simulink library "inp"  (R2021b)
settings: Solver=VariableStepAuto  StartTime=0.0  StopTime=10.0  RelTol=1e-3
undefined symbols (not defined in the file): C_TASK_5MS_S, FALSE, KINP_AcoreReadyToSlp_flg_ovrdflg, KINP_AcoreReadyToSlp_flg_ovrdval, KINP_AllowMovThd_OTA_enum_ovrdflg, KINP_AllowMovThd_OTA_enum_ovrdval, KINP_APSAngleTarget_Deg_ovrdflg, KINP_APSAngleTarget_Deg_ovrdval, KINP_APSDecReq_mps2_ovrdflg, KINP_APSDecReq_mps2_ovrdval, KINP_APSDecReqA_flg_ovrdflg, KINP_APSDecReqA_flg_ovrdval, KINP_APSDFLL_cm_ovrdflg, KINP_APSDFLL_cm_ovrdval, KINP_APSDFLR_cm_ovrdflg, KINP_APSDFLR_cm_ovrdval, KINP_APSDRLL_cm_ovrdflg, KINP_APSDRLL_cm_ovrdval, KINP_APSDRLR_cm_ovrdflg, KINP_APSDRLR_cm_ovrdval, KINP_APSExitCondition_enum_ovrdflg, KINP_APSExitCondition_enum_ovrdval, KINP_APSHWVer_enum_ovrdflg, KINP_APSHWVer_enum_ovrdval, KINP_APSProgressPCT_pct_ovrdflg, KINP_APSProgressPCT_pct_ovrdval, KINP_APSPwrReq_enum_ovrdflg, KINP_APSPwrReq_enum_ovrdval, KINP_APSReq_enum_ovrdflg, KINP_APSReq_enum_ovrdval, KINP_APSRQDisplay_enum_ovrdflg, KINP_APSRQDisplay_enum_ovrdval, KINP_APSRqEPASCtrl_flg_ovrdflg, KINP_APSRqEPASCtrl_flg_ovrdval, KINP_APSShiftPosnReq_enum_ovrdval, KINP_APSShiftPosnReq_enum_ovrflg, KINP_APSSpeedCMD_kph_ovrdval, KINP_APSSpeedCMD_kph_ovrflg, KINP_APSStaSystem_enum_ovrdflg, KINP_APSStaSystem_enum_ovrdval, KINP_APSSWVer_enum_ovrdflg, KINP_APSSWVer_enum_ovrdval, KINP_APSVMCReqA_flg_ovrdval, KINP_APSVMCReqA_flg_ovrflg, KINP_APSVRqEPASCtrl_flg_ovrdflg, KINP_APSVRqEPASCtrl_flg_ovrdval, KINP_AuxBattVolmV_mV_ovrdflg, KINP_AuxBattVolmV_mV_ovrdval, KINP_CAASSta_enum_ovrdflg, KINP_CAASSta_enum_ovrdval, KINP_CAASVMCReqA_flg_ovrdval, KINP_CAASVMCReqA_flg_ovrflg, KINP_CAN1BusOff_flg_ovrdflg, KINP_CAN1BusOff_flg_ovrdval, KINP_CAN2BusOff_flg_ovrdflg, KINP_CAN2BusOff_flg_ovrdval, KINP_CAN3BusOff_flg_ovrdflg, KINP_CAN3BusOff_flg_ovrdval, KINP_CAN4BusOff_flg_ovrdflg, KINP_CAN4BusOff_flg_ovrdval ... (+152)
libraries: FVT_lib x1035, hcu_lib x1
(part 23 of 33)

== system inp/INP/CAN3/SignalCheck/MCU_N_R1 ==
  BHAL_outputs : Inport
  inp_CanValid_bus : Inport  Port=2
  MCUNR1CSErr : FVT_lib/inp/can_signal_template  SystemSampleTime=-1  VariantActivationTime=update diagram  Latency=0  AutoFrameSizeCalculation=off
      link override defval: Value=KINP_MCUNR1CSErr_flg_defval
      link override ovrdflg: Value=KINP_MCUNR1CSErr_flg_ovrdflg
      link override ovrdval: Value=KINP_MCUNR1CSErr_flg_ovrdval
  MCUNR1RCErr : FVT_lib/inp/can_signal_template  SystemSampleTime=-1  VariantActivationTime=update diagram  Latency=0  AutoFrameSizeCalculation=off
      link override defval: Value=KINP_MCUNR1RCErr_flg_defval
      link override ovrdflg: Value=KINP_MCUNR1RCErr_flg_ovrdflg
      link override ovrdval: Value=KINP_MCUNR1RCErr_flg_ovrdval
  MCUWarnRNidec : FVT_lib/inp/can_signal_template  SystemSampleTime=-1  VariantActivationTime=update diagram  Latency=0  AutoFrameSizeCalculation=off
      link override defval: Value=KINP_MCUWarnRNidec_enum_defval
      link override ovrdflg: Value=KINP_MCUWarnRNidec_enum_ovrdflg
      link override ovrdval: Value=KINP_MCUWarnRNidec_enum_ovrdval
  RrActvDmpDisabStaNidec : FVT_lib/inp/can_signal_template  SystemSampleTime=-1  VariantActivationTime=update diagram  Latency=0  AutoFrameSizeCalculation=off
      link override defval: Value=KINP_RrActvDmpDisabStaNidec_flg_defval
      link override ovrdflg: Value=KINP_RrActvDmpDisabStaNidec_flg_ovrdflg
      link override ovrdval: Value=KINP_RrActvDmpDisabStaNidec_flg_ovrdval
  RrEDUDrtStaNidec : FVT_lib/inp/can_signal_template  SystemSampleTime=-1  VariantActivationTime=update diagram  Latency=0  AutoFrameSizeCalculation=off
      link override defval: Value=KINP_RrEDUDrtStaNidec_flg_defval
      link override ovrdflg: Value=KINP_RrEDUDrtStaNidec_flg_ovrdflg
      link override ovrdval: Value=KINP_RrEDUDrtStaNidec_flg_ovrdval
  RrEDUOpratingStaNidec : FVT_lib/inp/can_signal_template  SystemSampleTime=-1  VariantActivationTime=update diagram  Latency=0  AutoFrameSizeCalculation=off
      link override defval: Value=KINP_RrEDUOpratingStaNidec_flg_defval
      link override ovrdflg: Value=KINP_RrEDUOpratingStaNidec_flg_ovrdflg
      link override ovrdval: Value=KINP_RrEDUOpratingStaNidec_flg_ovrdval
  RrEDURealTMTqNidec : FVT_lib/inp/can_signal_template  SystemSampleTime=-1  VariantActivationTime=update diagram  Latency=0  AutoFrameSizeCalculation=off
      link override defval: Value=KINP_RrEDURealTMTqNidec_Nm_defval
      link override ovrdflg: Value=KINP_RrEDURealTMTqNidec_Nm_ovrdflg
      link override ovrdval: Value=KINP_RrEDURealTMTqNidec_Nm_ovrdval
  RrEDURotateDirctionNidec : FVT_lib/inp/can_signal_template  SystemSampleTime=-1  VariantActivationTime=update diagram  Latency=0  AutoFrameSizeCalculation=off
      link override defval: Value=KINP_RrEDURotateDirctionNidec_enum_defval
      link override ovrdflg: Value=KINP_RrEDURotateDirctionNidec_enum_ovrdflg
      link override ovrdval: Value=KINP_RrEDURotateDirctionNidec_enum_ovrdval
  RrEDUTqReqFbkNidec : FVT_lib/inp/can_signal_template  SystemSampleTime=-1  VariantActivationTime=update diagram  Latency=0  AutoFrameSizeCalculation=off
      link override defval: Value=KINP_RrEDUTqReqFbkNidec_Nm_defval
      link override ovrdflg: Value=KINP_RrEDUTqReqFbkNidec_Nm_ovrdflg
      link override ovrdval: Value=KINP_RrEDUTqReqFbkNidec_Nm_ovrdval
  RrMCU1ChksumNidec : FVT_lib/inp/can_signal_template  SystemSampleTime=-1  VariantActivationTime=update diagram  Latency=0  AutoFrameSizeCalculation=off
      link override defval: Value=KINP_RrMCU1ChksumNidec_enum_defval
      link override ovrdflg: Value=KINP_RrMCU1ChksumNidec_enum_ovrdflg
      link override ovrdval: Value=KINP_RrMCU1ChksumNidec_enum_ovrdval
  RrMCU1RolCntNidec : FVT_lib/inp/can_signal_template  SystemSampleTime=-1  VariantActivationTime=update diagram  Latency=0  AutoFrameSizeCalculation=off
      link override defval: Value=KINP_RrMCU1RolCntNidec_enum_defval
      link override ovrdflg: Value=KINP_RrMCU1RolCntNidec_enum_ovrdflg
      link override ovrdval: Value=KINP_RrMCU1RolCntNidec_enum_ovrdval
  RrMCUBATNidec : FVT_lib/inp/can_signal_template  SystemSampleTime=-1  VariantActivationTime=update diagram  Latency=0  AutoFrameSizeCalculation=off
      link override defval: Value=KINP_RrMCUBATNidec_V_defval
      link override ovrdflg: Value=KINP_RrMCUBATNidec_V_ovrdflg
      link override ovrdval: Value=KINP_RrMCUBATNidec_V_ovrdval
  RrMCUDCBusCurrNidec : FVT_lib/inp/can_signal_template  SystemSampleTime=-1  VariantActivationTime=update diagram  Latency=0  AutoFrameSizeCalculation=off
      link override defval: Value=KINP_RrMCUDCBusCurrNidec_A_defval
      link override ovrdflg: Value=KINP_RrMCUDCBusCurrNidec_A_ovrdflg
      link override ovrdval: Value=KINP_RrMCUDCBusCurrNidec_A_ovrdval
  RrMCUDCBusVoltNidec : FVT_lib/inp/can_signal_template  SystemSampleTime=-1  VariantActivationTime=update diagram  Latency=0  AutoFrameSizeCalculation=off
      link override defval: Value=KINP_RrMCUDCBusVoltNidec_V_defval
      link override ovrdflg: Value=KINP_RrMCUDCBusVoltNidec_V_ovrdflg
      link override ovrdval: Value=KINP_RrMCUDCBusVoltNidec_V_ovrdval
  RrMCUDischrgStaNidec : FVT_lib/inp/can_signal_template  SystemSampleTime=-1  VariantActivationTime=update diagram  Latency=0  AutoFrameSizeCalculation=off
      link override defval: Value=KINP_RrMCUDischrgStaNidec_flg_defval
      link override ovrdflg: Value=KINP_RrMCUDischrgStaNidec_flg_ovrdflg
      link override ovrdval: Value=KINP_RrMCUDischrgStaNidec_flg_ovrdval
  RrMCUEnaStaNidec : FVT_lib/inp/can_signal_template  SystemSampleTime=-1  VariantActivationTime=update diagram  Latency=0  AutoFrameSizeCalculation=off
      link override defval: Value=KINP_RrMCUEnaStaNidec_flg_defval
      link override ovrdflg: Value=KINP_RrMCUEnaStaNidec_flg_ovrdflg
      link override ovrdval: Value=KINP_RrMCUEnaStaNidec_flg_ovrdval
  RrMCUErrNidec : FVT_lib/inp/can_signal_template  SystemSampleTime=-1  VariantActivationTime=update diagram  Latency=0  AutoFrameSizeCalculation=off
      link override defval: Value=KINP_RrMCUErrNidec_enum_defval
      link override ovrdflg: Value=KINP_RrMCUErrNidec_enum_ovrdflg
      link override ovrdval: Value=KINP_RrMCUErrNidec_enum_ovrdval
  RrMCUIGNstaNidec : FVT_lib/inp/can_signal_template  SystemSampleTime=-1  VariantActivationTime=update diagram  Latency=0  AutoFrameSizeCalculation=off
      link override defval: Value=KINP_RrMCUIGNstaNidec_flg_defval
      link override ovrdflg: Value=KINP_RrMCUIGNstaNidec_flg_ovrdflg
      link override ovrdval: Value=KINP_RrMCUIGNstaNidec_flg_ovrdval
  RrMCUReady4PreNidec : FVT_lib/inp/can_signal_template  SystemSampleTime=-1  VariantActivationTime=update diagram  Latency=0  AutoFrameSizeCalculation=off
      link override defval: Value=KINP_RrMCUReady4PreNidec_flg_defval
      link override ovrdflg: Value=KINP_RrMCUReady4PreNidec_flg_ovrdflg
      link override ovrdval: Value=KINP_RrMCUReady4PreNidec_flg_ovrdval
  RrMCUReadyNidec : FVT_lib/inp/can_signal_template  SystemSampleTime=-1  VariantActivationTime=update diagram  Latency=0  AutoFrameSizeCalculation=off
      link override defval: Value=KINP_RrMCUReadyNidec_flg_defval
      link override ovrdflg: Value=KINP_RrMCUReadyNidec_flg_ovrdflg
      link override ovrdval: Value=KINP_RrMCUReadyNidec_flg_ovrdval
  RrMCUSysStaNidec : FVT_lib/inp/can_signal_template  SystemSampleTime=-1  VariantActivationTime=update diagram  Latency=0  AutoFrameSizeCalculation=off
      link override defval: Value=KINP_RrMCUSysStaNidec_enum_defval
      link override ovrdflg: Value=KINP_RrMCUSysStaNidec_enum_ovrdflg
      link override ovrdval: Value=KINP_RrMCUSysStaNidec_enum_ovrdval
  RrMCUTempNidec : FVT_lib/inp/can_signal_template  SystemSampleTime=-1  VariantActivationTime=update diagram  Latency=0  AutoFrameSizeCalculation=off
      link override defval: Value=KINP_RrMCUTempNidec_C_defval
      link override ovrdflg: Value=KINP_RrMCUTempNidec_C_ovrdflg
      link override ovrdval: Value=KINP_RrMCUTempNidec_C_ovrdval
  RrMotorAvailTqNidec : FVT_lib/inp/can_signal_template  SystemSampleTime=-1  VariantActivationTime=update diagram  Latency=0  AutoFrameSizeCalculation=off
      link override defval: Value=KINP_RrMotorAvailTqNidec_Nm_defval
      link override ovrdflg: Value=KINP_RrMotorAvailTqNidec_Nm_ovrdflg
      link override ovrdval: Value=KINP_RrMotorAvailTqNidec_Nm_ovrdval
  RrRegenAvailTqNidec : FVT_lib/inp/can_signal_template  SystemSampleTime=-1  VariantActivationTime=update diagram  Latency=0  AutoFrameSizeCalculation=off
      link override defval: Value=KINP_RrRegenAvailTqNidec_Nm_defval
      link override ovrdflg: Value=KINP_RrRegenAvailTqNidec_Nm_ovrdflg
      link override ovrdval: Value=KINP_RrRegenAvailTqNidec_Nm_ovrdval
  RrTMSpdNidec : FVT_lib/inp/can_signal_template  SystemSampleTime=-1  VariantActivationTime=update diagram  Latency=0  AutoFrameSizeCalculation=off
      link override defval: Value=KINP_RrTMSpdNidec_rpm_defval
      link override ovrdflg: Value=KINP_RrTMSpdNidec_rpm_ovrdflg
      link override ovrdval: Value=KINP_RrTMSpdNidec_rpm_ovrdval
  RrTMTempNidec : FVT_lib/inp/can_signal_template  SystemSampleTime=-1  VariantActivationTime=update diagram  Latency=0  AutoFrameSizeCalculation=off
      link override defval: Value=KINP_RrTMTempNidec_C_defval
      link override ovrdflg: Value=KINP_RrTMTempNidec_C_ovrdflg
      link override ovrdval: Value=KINP_RrTMTempNidec_C_ovrdval
  RrTMidNidec : FVT_lib/inp/can_signal_template  SystemSampleTime=-1  VariantActivationTime=update diagram  Latency=0  AutoFrameSizeCalculation=off
      link override defval: Value=KINP_RrTMidNidec_A_defval
      link override ovrdflg: Value=KINP_RrTMidNidec_A_ovrdflg
      link override ovrdval: Value=KINP_RrTMidNidec_A_ovrdval
  RrTMiqNidec : FVT_lib/inp/can_signal_template  SystemSampleTime=-1  VariantActivationTime=update diagram  Latency=0  AutoFrameSizeCalculation=off
      link override defval: Value=KINP_RrTMiqNidec_A_defval
      link override ovrdflg: Value=KINP_RrTMiqNidec_A_ovrdflg
      link override ovrdval: Value=KINP_RrTMiqNidec_A_ovrdval
  Terminator_{1..28} (28 alike) : Terminator
  True_VHAL_MCUNR1CSErr_flg : Constant  Value=TRUE  OutDataTypeStr=boolean
  True_VHAL_MCUNR1RCErr_flg : Constant  Value=TRUE  OutDataTypeStr=boolean
  True_VHAL_MCUWarnRNidec_enum : Constant  Value=TRUE  OutDataTypeStr=boolean
  True_VHAL_RrActvDmpDisabStaNidec_flg : Constant  Value=TRUE  OutDataTypeStr=boolean
  True_VHAL_RrEDUDrtStaNidec_flg : Constant  Value=TRUE  OutDataTypeStr=boolean
  True_VHAL_RrEDUOpratingStaNidec_flg : Constant  Value=TRUE  OutDataTypeStr=boolean
  True_VHAL_RrEDURealTMTqNidec_Nm : Constant  Value=TRUE  OutDataTypeStr=boolean
  True_VHAL_RrEDURotateDirctionNidec_enum : Constant  Value=TRUE  OutDataTypeStr=boolean
  True_VHAL_RrEDUTqReqFbkNidec_Nm : Constant  Value=TRUE  OutDataTypeStr=boolean
  True_VHAL_RrMCU1ChksumNidec_enum : Constant  Value=TRUE  OutDataTypeStr=boolean
  True_VHAL_RrMCU1RolCntNidec_enum : Constant  Value=TRUE  OutDataTypeStr=boolean
  True_VHAL_RrMCUBATNidec_V : Constant  Value=TRUE  OutDataTypeStr=boolean
  True_VHAL_RrMCUDCBusCurrNidec_A : Constant  Value=TRUE  OutDataTypeStr=boolean
  True_VHAL_RrMCUDCBusVoltNidec_V : Constant  Value=TRUE  OutDataTypeStr=boolean
  True_VHAL_RrMCUDischrgStaNidec_flg : Constant  Value=TRUE  OutDataTypeStr=boolean
  True_VHAL_RrMCUEnaStaNidec_flg : Constant  Value=TRUE  OutDataTypeStr=boolean
  True_VHAL_RrMCUErrNidec_enum : Constant  Value=TRUE  OutDataTypeStr=boolean
  True_VHAL_RrMCUIGNstaNidec_flg : Constant  Value=TRUE  OutDataTypeStr=boolean
  True_VHAL_RrMCUReady4PreNidec_flg : Constant  Value=TRUE  OutDataTypeStr=boolean
  True_VHAL_RrMCUReadyNidec_flg : Constant  Value=TRUE  OutDataTypeStr=boolean
  True_VHAL_RrMCUSysStaNidec_enum : Constant  Value=TRUE  OutDataTypeStr=boolean
  True_VHAL_RrMCUTempNidec_C : Constant  Value=TRUE  OutDataTypeStr=boolean
  True_VHAL_RrMotorAvailTqNidec_Nm : Constant  Value=TRUE  OutDataTypeStr=boolean
  True_VHAL_RrRegenAvailTqNidec_Nm : Constant  Value=TRUE  OutDataTypeStr=boolean
  True_VHAL_RrTMSpdNidec_rpm : Constant  Value=TRUE  OutDataTypeStr=boolean
  True_VHAL_RrTMTempNidec_C : Constant  Value=TRUE  OutDataTypeStr=boolean
  True_VHAL_RrTMidNidec_A : Constant  Value=TRUE  OutDataTypeStr=boolean
  True_VHAL_RrTMiqNidec_A : Constant  Value=TRUE  OutDataTypeStr=boolean
  slr1_{1..28} (28 alike) : BusSelector  OutputSignals=VINP_CANMsgValidMCUNR1_flg
  slr_VHAL_MCUNR1CSErr_flg : BusSelector  OutputSignals=VHAL_MCUNR1CSErr_flg
  slr_VHAL_MCUNR1RCErr_flg : BusSelector  OutputSignals=VHAL_MCUNR1RCErr_flg
  slr_VHAL_MCUWarnRNidec_enum : BusSelector  OutputSignals=VHAL_MCUWarnRNidec_enum
  slr_VHAL_RrActvDmpDisabStaNidec_flg : BusSelector  OutputSignals=VHAL_RrActvDmpDisabStaNidec_flg
  slr_VHAL_RrEDUDrtStaNidec_flg : BusSelector  OutputSignals=VHAL_RrEDUDrtStaNidec_flg
  slr_VHAL_RrEDUOpratingStaNidec_flg : BusSelector  OutputSignals=VHAL_RrEDUOpratingStaNidec_flg
  slr_VHAL_RrEDURealTMTqNidec_Nm : BusSelector  OutputSignals=VHAL_RrEDURealTMTqNidec_Nm
  slr_VHAL_RrEDURotateDirctionNidec_enum : BusSelector  OutputSignals=VHAL_RrEDURotateDirctionNidec_enum
  slr_VHAL_RrEDUTqReqFbkNidec_Nm : BusSelector  OutputSignals=VHAL_RrEDUTqReqFbkNidec_Nm
  slr_VHAL_RrMCU1ChksumNidec_enum : BusSelector  OutputSignals=VHAL_RrMCU1ChksumNidec_enum
  slr_VHAL_RrMCU1RolCntNidec_enum : BusSelector  OutputSignals=VHAL_RrMCU1RolCntNidec_enum
  slr_VHAL_RrMCUBATNidec_V : BusSelector  OutputSignals=VHAL_RrMCUBATNidec_V
  slr_VHAL_RrMCUDCBusCurrNidec_A : BusSelector  OutputSignals=VHAL_RrMCUDCBusCurrNidec_A
  slr_VHAL_RrMCUDCBusVoltNidec_V : BusSelector  OutputSignals=VHAL_RrMCUDCBusVoltNidec_V
  slr_VHAL_RrMCUDischrgStaNidec_flg : BusSelector  OutputSignals=VHAL_RrMCUDischrgStaNidec_flg
  slr_VHAL_RrMCUEnaStaNidec_flg : BusSelector  OutputSignals=VHAL_RrMCUEnaStaNidec_flg
  slr_VHAL_RrMCUErrNidec_enum : BusSelector  OutputSignals=VHAL_RrMCUErrNidec_enum
  slr_VHAL_RrMCUIGNstaNidec_flg : BusSelector  OutputSignals=VHAL_RrMCUIGNstaNidec_flg
  slr_VHAL_RrMCUReady4PreNidec_flg : BusSelector  OutputSignals=VHAL_RrMCUReady4PreNidec_flg
  slr_VHAL_RrMCUReadyNidec_flg : BusSelector  OutputSignals=VHAL_RrMCUReadyNidec_flg
  slr_VHAL_RrMCUSysStaNidec_enum : BusSelector  OutputSignals=VHAL_RrMCUSysStaNidec_enum
  slr_VHAL_RrMCUTempNidec_C : BusSelector  OutputSignals=VHAL_RrMCUTempNidec_C
  slr_VHAL_RrMotorAvailTqNidec_Nm : BusSelector  OutputSignals=VHAL_RrMotorAvailTqNidec_Nm
  slr_VHAL_RrRegenAvailTqNidec_Nm : BusSelector  OutputSignals=VHAL_RrRegenAvailTqNidec_Nm
  slr_VHAL_RrTMSpdNidec_rpm : BusSelector  OutputSignals=VHAL_RrTMSpdNidec_rpm
  slr_VHAL_RrTMTempNidec_C : BusSelector  OutputSignals=VHAL_RrTMTempNidec_C
  slr_VHAL_RrTMidNidec_A : BusSelector  OutputSignals=VHAL_RrTMidNidec_A
  slr_VHAL_RrTMiqNidec_A : BusSelector  OutputSignals=VHAL_RrTMiqNidec_A
  VINP_MCUNR1CSErr_flg : Outport
  VINP_MCUNR1RCErr_flg : Outport  Port=2
  VINP_MCUWarnRNidec_enum : Outport  Port=3
  VINP_RrActvDmpDisabStaNidec_flg : Outport  Port=4
  VINP_RrEDUDrtStaNidec_flg : Outport  Port=5
  VINP_RrEDUOpratingStaNidec_flg : Outport  Port=6
  VINP_RrEDURealTMTqNidec_Nm : Outport  Port=7
  VINP_RrEDURotateDirctionNidec_enum : Outport  Port=8
  VINP_RrEDUTqReqFbkNidec_Nm : Outport  Port=9
  VINP_RrMCU1ChksumNidec_enum : Outport  Port=10
  VINP_RrMCU1RolCntNidec_enum : Outport  Port=11
  VINP_RrMCUBATNidec_V : Outport  Port=12
  VINP_RrMCUDCBusCurrNidec_A : Outport  Port=13
  VINP_RrMCUDCBusVoltNidec_V : Outport  Port=14
  VINP_RrMCUDischrgStaNidec_flg : Outport  Port=15
  VINP_RrMCUEnaStaNidec_flg : Outport  Port=16
  VINP_RrMCUErrNidec_enum : Outport  Port=17
  VINP_RrMCUIGNstaNidec_flg : Outport  Port=18
  VINP_RrMCUReady4PreNidec_flg : Outport  Port=19
  VINP_RrMCUReadyNidec_flg : Outport  Port=20
  VINP_RrMCUSysStaNidec_enum : Outport  Port=21
  VINP_RrMCUTempNidec_C : Outport  Port=22
  VINP_RrMotorAvailTqNidec_Nm : Outport  Port=23
  VINP_RrRegenAvailTqNidec_Nm : Outport  Port=24
  VINP_RrTMSpdNidec_rpm : Outport  Port=25
  VINP_RrTMTempNidec_C : Outport  Port=26
  VINP_RrTMidNidec_A : Outport  Port=27
  VINP_RrTMiqNidec_A : Outport  Port=28
  wires:
  BHAL_outputs/1 -> [BHAL_outputs]
  inp_CanValid_bus/1 -> [inp_CanValid_bus]
  [BHAL_outputs] -> slr_VHAL_MCUNR1CSErr_flg/1
  slr_VHAL_MCUNR1CSErr_flg/1 -> MCUNR1CSErr/1  "<VHAL_MCUNR1CSErr_flg>"
  True_VHAL_MCUNR1CSErr_flg/1 -> MCUNR1CSErr/2
  [inp_CanValid_bus] -> slr1_1/1
  slr1_1/1 -> MCUNR1CSErr/3  "<VINP_CANMsgValidMCUNR1_flg>"
  MCUNR1CSErr/1 -> VINP_MCUNR1CSErr_flg/1  "VINP_MCUNR1CSErr_flg"
  MCUNR1CSErr/2 -> Terminator_1/1
  [BHAL_outputs] -> slr_VHAL_MCUNR1RCErr_flg/1
  slr_VHAL_MCUNR1RCErr_flg/1 -> MCUNR1RCErr/1  "<VHAL_MCUNR1RCErr_flg>"
  True_VHAL_MCUNR1RCErr_flg/1 -> MCUNR1RCErr/2
  [inp_CanValid_bus] -> slr1_2/1
  slr1_2/1 -> MCUNR1RCErr/3  "<VINP_CANMsgValidMCUNR1_flg>"
  MCUNR1RCErr/1 -> VINP_MCUNR1RCErr_flg/1  "VINP_MCUNR1RCErr_flg"
  MCUNR1RCErr/2 -> Terminator_2/1
  [BHAL_outputs] -> slr_VHAL_MCUWarnRNidec_enum/1
  slr_VHAL_MCUWarnRNidec_enum/1 -> MCUWarnRNidec/1  "<VHAL_MCUWarnRNidec_enum>"
  True_VHAL_MCUWarnRNidec_enum/1 -> MCUWarnRNidec/2
  [inp_CanValid_bus] -> slr1_3/1
  slr1_3/1 -> MCUWarnRNidec/3  "<VINP_CANMsgValidMCUNR1_flg>"
  MCUWarnRNidec/1 -> VINP_MCUWarnRNidec_enum/1  "VINP_MCUWarnRNidec_enum"
  MCUWarnRNidec/2 -> Terminator_3/1
  [BHAL_outputs] -> slr_VHAL_RrActvDmpDisabStaNidec_flg/1
  slr_VHAL_RrActvDmpDisabStaNidec_flg/1 -> RrActvDmpDisabStaNidec/1  "<VHAL_RrActvDmpDisabStaNidec_flg>"
  True_VHAL_RrActvDmpDisabStaNidec_flg/1 -> RrActvDmpDisabStaNidec/2
  [inp_CanValid_bus] -> slr1_4/1
  slr1_4/1 -> RrActvDmpDisabStaNidec/3  "<VINP_CANMsgValidMCUNR1_flg>"
  RrActvDmpDisabStaNidec/1 -> VINP_RrActvDmpDisabStaNidec_flg/1  "VINP_RrActvDmpDisabStaNidec_flg"
  RrActvDmpDisabStaNidec/2 -> Terminator_4/1
  [BHAL_outputs] -> slr_VHAL_RrEDUDrtStaNidec_flg/1
  slr_VHAL_RrEDUDrtStaNidec_flg/1 -> RrEDUDrtStaNidec/1  "<VHAL_RrEDUDrtStaNidec_flg>"
  True_VHAL_RrEDUDrtStaNidec_flg/1 -> RrEDUDrtStaNidec/2
  [inp_CanValid_bus] -> slr1_5/1
  slr1_5/1 -> RrEDUDrtStaNidec/3  "<VINP_CANMsgValidMCUNR1_flg>"
  RrEDUDrtStaNidec/1 -> VINP_RrEDUDrtStaNidec_flg/1  "VINP_RrEDUDrtStaNidec_flg"
  RrEDUDrtStaNidec/2 -> Terminator_5/1
  [BHAL_outputs] -> slr_VHAL_RrEDUOpratingStaNidec_flg/1
  slr_VHAL_RrEDUOpratingStaNidec_flg/1 -> RrEDUOpratingStaNidec/1  "<VHAL_RrEDUOpratingStaNidec_flg>"
  True_VHAL_RrEDUOpratingStaNidec_flg/1 -> RrEDUOpratingStaNidec/2
  [inp_CanValid_bus] -> slr1_6/1
  slr1_6/1 -> RrEDUOpratingStaNidec/3  "<VINP_CANMsgValidMCUNR1_flg>"
  RrEDUOpratingStaNidec/1 -> VINP_RrEDUOpratingStaNidec_flg/1  "VINP_RrEDUOpratingStaNidec_flg"
  RrEDUOpratingStaNidec/2 -> Terminator_6/1
  [BHAL_outputs] -> slr_VHAL_RrEDURealTMTqNidec_Nm/1
  slr_VHAL_RrEDURealTMTqNidec_Nm/1 -> RrEDURealTMTqNidec/1  "<VHAL_RrEDURealTMTqNidec_Nm>"
  True_VHAL_RrEDURealTMTqNidec_Nm/1 -> RrEDURealTMTqNidec/2
  [inp_CanValid_bus] -> slr1_7/1
  slr1_7/1 -> RrEDURealTMTqNidec/3  "<VINP_CANMsgValidMCUNR1_flg>"
  RrEDURealTMTqNidec/1 -> VINP_RrEDURealTMTqNidec_Nm/1  "VINP_RrEDURealTMTqNidec_Nm"
  RrEDURealTMTqNidec/2 -> Terminator_7/1
  [BHAL_outputs] -> slr_VHAL_RrEDURotateDirctionNidec_enum/1
  slr_VHAL_RrEDURotateDirctionNidec_enum/1 -> RrEDURotateDirctionNidec/1  "<VHAL_RrEDURotateDirctionNidec_enum>"
  True_VHAL_RrEDURotateDirctionNidec_enum/1 -> RrEDURotateDirctionNidec/2
  [inp_CanValid_bus] -> slr1_8/1
  slr1_8/1 -> RrEDURotateDirctionNidec/3  "<VINP_CANMsgValidMCUNR1_flg>"
  RrEDURotateDirctionNidec/1 -> VINP_RrEDURotateDirctionNidec_enum/1  "VINP_RrEDURotateDirctionNidec_enum"
  RrEDURotateDirctionNidec/2 -> Terminator_8/1
  [BHAL_outputs] -> slr_VHAL_RrEDUTqReqFbkNidec_Nm/1
  slr_VHAL_RrEDUTqReqFbkNidec_Nm/1 -> RrEDUTqReqFbkNidec/1  "<VHAL_RrEDUTqReqFbkNidec_Nm>"
  True_VHAL_RrEDUTqReqFbkNidec_Nm/1 -> RrEDUTqReqFbkNidec/2
  [inp_CanValid_bus] -> slr1_9/1
  slr1_9/1 -> RrEDUTqReqFbkNidec/3  "<VINP_CANMsgValidMCUNR1_flg>"
  RrEDUTqReqFbkNidec/1 -> VINP_RrEDUTqReqFbkNidec_Nm/1  "VINP_RrEDUTqReqFbkNidec_Nm"
  RrEDUTqReqFbkNidec/2 -> Terminator_9/1
  [BHAL_outputs] -> slr_VHAL_RrMCU1ChksumNidec_enum/1
  slr_VHAL_RrMCU1ChksumNidec_enum/1 -> RrMCU1ChksumNidec/1  "<VHAL_RrMCU1ChksumNidec_enum>"
  True_VHAL_RrMCU1ChksumNidec_enum/1 -> RrMCU1ChksumNidec/2
  [inp_CanValid_bus] -> slr1_10/1
  slr1_10/1 -> RrMCU1ChksumNidec/3  "<VINP_CANMsgValidMCUNR1_flg>"
  RrMCU1ChksumNidec/1 -> VINP_RrMCU1ChksumNidec_enum/1  "VINP_RrMCU1ChksumNidec_enum"
  RrMCU1ChksumNidec/2 -> Terminator_10/1
  [BHAL_outputs] -> slr_VHAL_RrMCU1RolCntNidec_enum/1
  slr_VHAL_RrMCU1RolCntNidec_enum/1 -> RrMCU1RolCntNidec/1  "<VHAL_RrMCU1RolCntNidec_enum>"
  True_VHAL_RrMCU1RolCntNidec_enum/1 -> RrMCU1RolCntNidec/2
  [inp_CanValid_bus] -> slr1_11/1
  slr1_11/1 -> RrMCU1RolCntNidec/3  "<VINP_CANMsgValidMCUNR1_flg>"
  RrMCU1RolCntNidec/1 -> VINP_RrMCU1RolCntNidec_enum/1  "VINP_RrMCU1RolCntNidec_enum"
  RrMCU1RolCntNidec/2 -> Terminator_11/1
  [BHAL_outputs] -> slr_VHAL_RrMCUBATNidec_V/1
  slr_VHAL_RrMCUBATNidec_V/1 -> RrMCUBATNidec/1  "<VHAL_RrMCUBATNidec_V>"
  True_VHAL_RrMCUBATNidec_V/1 -> RrMCUBATNidec/2
  [inp_CanValid_bus] -> slr1_12/1
  slr1_12/1 -> RrMCUBATNidec/3  "<VINP_CANMsgValidMCUNR1_flg>"
  RrMCUBATNidec/1 -> VINP_RrMCUBATNidec_V/1  "VINP_RrMCUBATNidec_V"
  RrMCUBATNidec/2 -> Terminator_12/1
  [BHAL_outputs] -> slr_VHAL_RrMCUDCBusCurrNidec_A/1
  slr_VHAL_RrMCUDCBusCurrNidec_A/1 -> RrMCUDCBusCurrNidec/1  "<VHAL_RrMCUDCBusCurrNidec_A>"
  True_VHAL_RrMCUDCBusCurrNidec_A/1 -> RrMCUDCBusCurrNidec/2
  [inp_CanValid_bus] -> slr1_13/1
  slr1_13/1 -> RrMCUDCBusCurrNidec/3  "<VINP_CANMsgValidMCUNR1_flg>"
  RrMCUDCBusCurrNidec/1 -> VINP_RrMCUDCBusCurrNidec_A/1  "VINP_RrMCUDCBusCurrNidec_A"
  RrMCUDCBusCurrNidec/2 -> Terminator_13/1
  [BHAL_outputs] -> slr_VHAL_RrMCUDCBusVoltNidec_V/1
  slr_VHAL_RrMCUDCBusVoltNidec_V/1 -> RrMCUDCBusVoltNidec/1  "<VHAL_RrMCUDCBusVoltNidec_V>"
  True_VHAL_RrMCUDCBusVoltNidec_V/1 -> RrMCUDCBusVoltNidec/2
  [inp_CanValid_bus] -> slr1_14/1
  slr1_14/1 -> RrMCUDCBusVoltNidec/3  "<VINP_CANMsgValidMCUNR1_flg>"
  RrMCUDCBusVoltNidec/1 -> VINP_RrMCUDCBusVoltNidec_V/1  "VINP_RrMCUDCBusVoltNidec_V"
  RrMCUDCBusVoltNidec/2 -> Terminator_14/1
  [BHAL_outputs] -> slr_VHAL_RrMCUDischrgStaNidec_flg/1
  slr_VHAL_RrMCUDischrgStaNidec_flg/1 -> RrMCUDischrgStaNidec/1  "<VHAL_RrMCUDischrgStaNidec_flg>"
  True_VHAL_RrMCUDischrgStaNidec_flg/1 -> RrMCUDischrgStaNidec/2
  [inp_CanValid_bus] -> slr1_15/1
  slr1_15/1 -> RrMCUDischrgStaNidec/3  "<VINP_CANMsgValidMCUNR1_flg>"
  RrMCUDischrgStaNidec/1 -> VINP_RrMCUDischrgStaNidec_flg/1  "VINP_RrMCUDischrgStaNidec_flg"
  RrMCUDischrgStaNidec/2 -> Terminator_15/1
  [BHAL_outputs] -> slr_VHAL_RrMCUEnaStaNidec_flg/1
  slr_VHAL_RrMCUEnaStaNidec_flg/1 -> RrMCUEnaStaNidec/1  "<VHAL_RrMCUEnaStaNidec_flg>"
  True_VHAL_RrMCUEnaStaNidec_flg/1 -> RrMCUEnaStaNidec/2
  [inp_CanValid_bus] -> slr1_16/1
  slr1_16/1 -> RrMCUEnaStaNidec/3  "<VINP_CANMsgValidMCUNR1_flg>"
  RrMCUEnaStaNidec/1 -> VINP_RrMCUEnaStaNidec_flg/1  "VINP_RrMCUEnaStaNidec_flg"
  RrMCUEnaStaNidec/2 -> Terminator_16/1
  [BHAL_outputs] -> slr_VHAL_RrMCUErrNidec_enum/1
  slr_VHAL_RrMCUErrNidec_enum/1 -> RrMCUErrNidec/1  "<VHAL_RrMCUErrNidec_enum>"
  True_VHAL_RrMCUErrNidec_enum/1 -> RrMCUErrNidec/2
  [inp_CanValid_bus] -> slr1_17/1
  slr1_17/1 -> RrMCUErrNidec/3  "<VINP_CANMsgValidMCUNR1_flg>"
  RrMCUErrNidec/1 -> VINP_RrMCUErrNidec_enum/1  "VINP_RrMCUErrNidec_enum"
  RrMCUErrNidec/2 -> Terminator_17/1
  [BHAL_outputs] -> slr_VHAL_RrMCUIGNstaNidec_flg/1
  slr_VHAL_RrMCUIGNstaNidec_flg/1 -> RrMCUIGNstaNidec/1  "<VHAL_RrMCUIGNstaNidec_flg>"
  True_VHAL_RrMCUIGNstaNidec_flg/1 -> RrMCUIGNstaNidec/2
  [inp_CanValid_bus] -> slr1_18/1
  slr1_18/1 -> RrMCUIGNstaNidec/3  "<VINP_CANMsgValidMCUNR1_flg>"
  RrMCUIGNstaNidec/1 -> VINP_RrMCUIGNstaNidec_flg/1  "VINP_RrMCUIGNstaNidec_flg"
  RrMCUIGNstaNidec/2 -> Terminator_18/1
  [BHAL_outputs] -> slr_VHAL_RrMCUReady4PreNidec_flg/1
  slr_VHAL_RrMCUReady4PreNidec_flg/1 -> RrMCUReady4PreNidec/1  "<VHAL_RrMCUReady4PreNidec_flg>"
  True_VHAL_RrMCUReady4PreNidec_flg/1 -> RrMCUReady4PreNidec/2
  [inp_CanValid_bus] -> slr1_19/1
  slr1_19/1 -> RrMCUReady4PreNidec/3  "<VINP_CANMsgValidMCUNR1_flg>"
  RrMCUReady4PreNidec/1 -> VINP_RrMCUReady4PreNidec_flg/1  "VINP_RrMCUReady4PreNidec_flg"
  RrMCUReady4PreNidec/2 -> Terminator_19/1
  [BHAL_outputs] -> slr_VHAL_RrMCUReadyNidec_flg/1
  slr_VHAL_RrMCUReadyNidec_flg/1 -> RrMCUReadyNidec/1  "<VHAL_RrMCUReadyNidec_flg>"
  True_VHAL_RrMCUReadyNidec_flg/1 -> RrMCUReadyNidec/2
  [inp_CanValid_bus] -> slr1_20/1
  slr1_20/1 -> RrMCUReadyNidec/3  "<VINP_CANMsgValidMCUNR1_flg>"
  RrMCUReadyNidec/1 -> VINP_RrMCUReadyNidec_flg/1  "VINP_RrMCUReadyNidec_flg"
  RrMCUReadyNidec/2 -> Terminator_20/1
  [BHAL_outputs] -> slr_VHAL_RrMCUSysStaNidec_enum/1
  slr_VHAL_RrMCUSysStaNidec_enum/1 -> RrMCUSysStaNidec/1  "<VHAL_RrMCUSysStaNidec_enum>"
  True_VHAL_RrMCUSysStaNidec_enum/1 -> RrMCUSysStaNidec/2
  [inp_CanValid_bus] -> slr1_21/1
  slr1_21/1 -> RrMCUSysStaNidec/3  "<VINP_CANMsgValidMCUNR1_flg>"
  RrMCUSysStaNidec/1 -> VINP_RrMCUSysStaNidec_enum/1  "VINP_RrMCUSysStaNidec_enum"
  RrMCUSysStaNidec/2 -> Terminator_21/1
  [BHAL_outputs] -> slr_VHAL_RrMCUTempNidec_C/1
  slr_VHAL_RrMCUTempNidec_C/1 -> RrMCUTempNidec/1  "<VHAL_RrMCUTempNidec_C>"
  True_VHAL_RrMCUTempNidec_C/1 -> RrMCUTempNidec/2
  [inp_CanValid_bus] -> slr1_22/1
  slr1_22/1 -> RrMCUTempNidec/3  "<VINP_CANMsgValidMCUNR1_flg>"
  RrMCUTempNidec/1 -> VINP_RrMCUTempNidec_C/1  "VINP_RrMCUTempNidec_C"
  RrMCUTempNidec/2 -> Terminator_22/1
  [BHAL_outputs] -> slr_VHAL_RrMotorAvailTqNidec_Nm/1
  slr_VHAL_RrMotorAvailTqNidec_Nm/1 -> RrMotorAvailTqNidec/1  "<VHAL_RrMotorAvailTqNidec_Nm>"
  True_VHAL_RrMotorAvailTqNidec_Nm/1 -> RrMotorAvailTqNidec/2
  [inp_CanValid_bus] -> slr1_23/1
  slr1_23/1 -> RrMotorAvailTqNidec/3  "<VINP_CANMsgValidMCUNR1_flg>"
  RrMotorAvailTqNidec/1 -> VINP_RrMotorAvailTqNidec_Nm/1  "VINP_RrMotorAvailTqNidec_Nm"
  RrMotorAvailTqNidec/2 -> Terminator_23/1
  [BHAL_outputs] -> slr_VHAL_RrRegenAvailTqNidec_Nm/1
  slr_VHAL_RrRegenAvailTqNidec_Nm/1 -> RrRegenAvailTqNidec/1  "<VHAL_RrRegenAvailTqNidec_Nm>"
  True_VHAL_RrRegenAvailTqNidec_Nm/1 -> RrRegenAvailTqNidec/2
  [inp_CanValid_bus] -> slr1_24/1
  slr1_24/1 -> RrRegenAvailTqNidec/3  "<VINP_CANMsgValidMCUNR1_flg>"
  RrRegenAvailTqNidec/1 -> VINP_RrRegenAvailTqNidec_Nm/1  "VINP_RrRegenAvailTqNidec_Nm"
  RrRegenAvailTqNidec/2 -> Terminator_24/1
  [BHAL_outputs] -> slr_VHAL_RrTMSpdNidec_rpm/1
  slr_VHAL_RrTMSpdNidec_rpm/1 -> RrTMSpdNidec/1  "<VHAL_RrTMSpdNidec_rpm>"
  True_VHAL_RrTMSpdNidec_rpm/1 -> RrTMSpdNidec/2
  [inp_CanValid_bus] -> slr1_25/1
  slr1_25/1 -> RrTMSpdNidec/3  "<VINP_CANMsgValidMCUNR1_flg>"
  RrTMSpdNidec/1 -> VINP_RrTMSpdNidec_rpm/1  "VINP_RrTMSpdNidec_rpm"
  RrTMSpdNidec/2 -> Terminator_25/1
  [BHAL_outputs] -> slr_VHAL_RrTMTempNidec_C/1
  slr_VHAL_RrTMTempNidec_C/1 -> RrTMTempNidec/1  "<VHAL_RrTMTempNidec_C>"
  True_VHAL_RrTMTempNidec_C/1 -> RrTMTempNidec/2
  [inp_CanValid_bus] -> slr1_26/1
  slr1_26/1 -> RrTMTempNidec/3  "<VINP_CANMsgValidMCUNR1_flg>"
  RrTMTempNidec/1 -> VINP_RrTMTempNidec_C/1  "VINP_RrTMTempNidec_C"
  RrTMTempNidec/2 -> Terminator_26/1
  [BHAL_outputs] -> slr_VHAL_RrTMidNidec_A/1
  slr_VHAL_RrTMidNidec_A/1 -> RrTMidNidec/1  "<VHAL_RrTMidNidec_A>"
  True_VHAL_RrTMidNidec_A/1 -> RrTMidNidec/2
  [inp_CanValid_bus] -> slr1_27/1
  slr1_27/1 -> RrTMidNidec/3  "<VINP_CANMsgValidMCUNR1_flg>"
  RrTMidNidec/1 -> VINP_RrTMidNidec_A/1  "VINP_RrTMidNidec_A"
  RrTMidNidec/2 -> Terminator_27/1
  [BHAL_outputs] -> slr_VHAL_RrTMiqNidec_A/1
  slr_VHAL_RrTMiqNidec_A/1 -> RrTMiqNidec/1  "<VHAL_RrTMiqNidec_A>"
  True_VHAL_RrTMiqNidec_A/1 -> RrTMiqNidec/2
  [inp_CanValid_bus] -> slr1_28/1
  slr1_28/1 -> RrTMiqNidec/3  "<VINP_CANMsgValidMCUNR1_flg>"
  RrTMiqNidec/1 -> VINP_RrTMiqNidec_A/1  "VINP_RrTMiqNidec_A"
  RrTMiqNidec/2 -> Terminator_28/1

== system inp/INP/CAN3/SignalCheck/MCU_N_R2 ==
  BHAL_outputs : Inport
  inp_CanValid_bus : Inport  Port=2
  RrCoolanttempReqNidec : FVT_lib/inp/can_signal_template  SystemSampleTime=-1  VariantActivationTime=update diagram  Latency=0  AutoFrameSizeCalculation=off
      link override defval: Value=KINP_RrCoolanttempReqNidec_cnt_defval
      link override ovrdflg: Value=KINP_RrCoolanttempReqNidec_cnt_ovrdflg
      link override ovrdval: Value=KINP_RrCoolanttempReqNidec_cnt_ovrdval
  RrEOPSpdSetNidec : FVT_lib/inp/can_signal_template  SystemSampleTime=-1  VariantActivationTime=update diagram  Latency=0  AutoFrameSizeCalculation=off
      link override defval: Value=KINP_RrEOPSpdSetNidec_rpm_defval
      link override ovrdflg: Value=KINP_RrEOPSpdSetNidec_rpm_ovrdflg
      link override ovrdval: Value=KINP_RrEOPSpdSetNidec_rpm_ovrdval
  RrFailcode1Nidec : FVT_lib/inp/can_signal_template  SystemSampleTime=-1  VariantActivationTime=update diagram  Latency=0  AutoFrameSizeCalculation=off
      link override defval: Value=KINP_RrFailcode1Nidec_enum_defval
      link override ovrdflg: Value=KINP_RrFailcode1Nidec_enum_ovrdflg
      link override ovrdval: Value=KINP_RrFailcode1Nidec_enum_ovrdval
  RrFailcode2Nidec : FVT_lib/inp/can_signal_template  SystemSampleTime=-1  VariantActivationTime=update diagram  Latency=0  AutoFrameSizeCalculation=off
      link override defval: Value=KINP_RrFailcode2Nidec_enum_defval
      link override ovrdflg: Value=KINP_RrFailcode2Nidec_enum_ovrdflg
      link override ovrdval: Value=KINP_RrFailcode2Nidec_enum_ovrdval
  RrFailcodehistory1Nidec : FVT_lib/inp/can_signal_template  SystemSampleTime=-1  VariantActivationTime=update diagram  Latency=0  AutoFrameSizeCalculation=off
      link override defval: Value=KINP_RrFailcodehistory1Nidec_enum_defval
      link override ovrdflg: Value=KINP_RrFailcodehistory1Nidec_enum_ovrdflg
      link override ovrdval: Value=KINP_RrFailcodehistory1Nidec_enum_ovrdval
  RrFailcodehistory2Nidec : FVT_lib/inp/can_signal_template  SystemSampleTime=-1  VariantActivationTime=update diagram  Latency=0  AutoFrameSizeCalculation=off
      link override defval: Value=KINP_RrFailcodehistory2Nidec_enum_defval
      link override ovrdflg: Value=KINP_RrFailcodehistory2Nidec_enum_ovrdflg
      link override ovrdval: Value=KINP_RrFailcodehistory2Nidec_enum_ovrdval
  RrLLCTempNidec : FVT_lib/inp/can_signal_template  SystemSampleTime=-1  VariantActivationTime=update diagram  Latency=0  AutoFrameSizeCalculation=off
      link override defval: Value=KINP_RrLLCTempNidec_C_defval
      link override ovrdflg: Value=KINP_RrLLCTempNidec_C_ovrdflg
      link override ovrdval: Value=KINP_RrLLCTempNidec_C_ovrdval
  RrLLCflowReqNidec : FVT_lib/inp/can_signal_template  SystemSampleTime=-1  VariantActivationTime=update diagram  Latency=0  AutoFrameSizeCalculation=off
      link override defval: Value=KINP_RrLLCflowReqNidec_Lpmin_defval
      link override ovrdflg: Value=KINP_RrLLCflowReqNidec_Lpmin_ovrdflg
      link override ovrdval: Value=KINP_RrLLCflowReqNidec_Lpmin_ovrdval
  RrMCUTempWarnNidec : FVT_lib/inp/can_signal_template  SystemSampleTime=-1  VariantActivationTime=update diagram  Latency=0  AutoFrameSizeCalculation=off
      link override defval: Value=KINP_RrMCUTempWarnNidec_enum_defval
      link override ovrdflg: Value=KINP_RrMCUTempWarnNidec_enum_ovrdflg
      link override ovrdval: Value=KINP_RrMCUTempWarnNidec_enum_ovrdval
  RrTMTempWarnNidec : FVT_lib/inp/can_signal_template  SystemSampleTime=-1  VariantActivationTime=update diagram  Latency=0  AutoFrameSizeCalculation=off
      link override defval: Value=KINP_RrTMTempWarnNidec_enum_defval
      link override ovrdflg: Value=KINP_RrTMTempWarnNidec_enum_ovrdflg
      link override ovrdval: Value=KINP_RrTMTempWarnNidec_enum_ovrdval
  Terminator_{1..10} (10 alike) : Terminator
  True_VHAL_RrCoolanttempReqNidec_cnt : Constant  Value=TRUE  OutDataTypeStr=boolean
  True_VHAL_RrEOPSpdSetNidec_rpm : Constant  Value=TRUE  OutDataTypeStr=boolean
  True_VHAL_RrFailcode1Nidec_enum : Constant  Value=TRUE  OutDataTypeStr=boolean
  True_VHAL_RrFailcode2Nidec_enum : Constant  Value=TRUE  OutDataTypeStr=boolean
  True_VHAL_RrFailcodehistory1Nidec_enum : Constant  Value=TRUE  OutDataTypeStr=boolean
  True_VHAL_RrFailcodehistory2Nidec_enum : Constant  Value=TRUE  OutDataTypeStr=boolean
  True_VHAL_RrLLCTempNidec_C : Constant  Value=TRUE  OutDataTypeStr=boolean
  True_VHAL_RrLLCflowReqNidec_Lpmin : Constant  Value=TRUE  OutDataTypeStr=boolean
  True_VHAL_RrMCUTempWarnNidec_enum : Constant  Value=TRUE  OutDataTypeStr=boolean
  True_VHAL_RrTMTempWarnNidec_enum : Constant  Value=TRUE  OutDataTypeStr=boolean
  slr1_{1..10} (10 alike) : BusSelector  OutputSignals=VINP_CANMsgValidMCUNR2_flg
  slr_VHAL_RrCoolanttempReqNidec_cnt : BusSelector  OutputSignals=VHAL_RrCoolanttempReqNidec_cnt
  slr_VHAL_RrEOPSpdSetNidec_rpm : BusSelector  OutputSignals=VHAL_RrEOPSpdSetNidec_rpm
  slr_VHAL_RrFailcode1Nidec_enum : BusSelector  OutputSignals=VHAL_RrFailcode1Nidec_enum
  slr_VHAL_RrFailcode2Nidec_enum : BusSelector  OutputSignals=VHAL_RrFailcode2Nidec_enum
  slr_VHAL_RrFailcodehistory1Nidec_enum : BusSelector  OutputSignals=VHAL_RrFailcodehistory1Nidec_enum
  slr_VHAL_RrFailcodehistory2Nidec_enum : BusSelector  OutputSignals=VHAL_RrFailcodehistory2Nidec_enum
  slr_VHAL_RrLLCTempNidec_C : BusSelector  OutputSignals=VHAL_RrLLCTempNidec_C
  slr_VHAL_RrLLCflowReqNidec_Lpmin : BusSelector  OutputSignals=VHAL_RrLLCflowReqNidec_Lpmin
  slr_VHAL_RrMCUTempWarnNidec_enum : BusSelector  OutputSignals=VHAL_RrMCUTempWarnNidec_enum
  slr_VHAL_RrTMTempWarnNidec_enum : BusSelector  OutputSignals=VHAL_RrTMTempWarnNidec_enum
  VINP_RrCoolanttempReqNidec_cnt : Outport
  VINP_RrEOPSpdSetNidec_rpm : Outport  Port=2
  VINP_RrFailcode1Nidec_enum : Outport  Port=3
  VINP_RrFailcode2Nidec_enum : Outport  Port=4
  VINP_RrFailcodehistory1Nidec_enum : Outport  Port=5
  VINP_RrFailcodehistory2Nidec_enum : Outport  Port=6
  VINP_RrLLCTempNidec_C : Outport  Port=7
  VINP_RrLLCflowReqNidec_Lpmin : Outport  Port=8
  VINP_RrMCUTempWarnNidec_enum : Outport  Port=9
  VINP_RrTMTempWarnNidec_enum : Outport  Port=10
  wires:
  BHAL_outputs/1 -> [BHAL_outputs]
  inp_CanValid_bus/1 -> [inp_CanValid_bus]
  [BHAL_outputs] -> slr_VHAL_RrCoolanttempReqNidec_cnt/1
  slr_VHAL_RrCoolanttempReqNidec_cnt/1 -> RrCoolanttempReqNidec/1  "<VHAL_RrCoolanttempReqNidec_cnt>"
  True_VHAL_RrCoolanttempReqNidec_cnt/1 -> RrCoolanttempReqNidec/2
  [inp_CanValid_bus] -> slr1_1/1
  slr1_1/1 -> RrCoolanttempReqNidec/3  "<VINP_CANMsgValidMCUNR2_flg>"
  RrCoolanttempReqNidec/1 -> VINP_RrCoolanttempReqNidec_cnt/1  "VINP_RrCoolanttempReqNidec_cnt"
  RrCoolanttempReqNidec/2 -> Terminator_1/1
  [BHAL_outputs] -> slr_VHAL_RrEOPSpdSetNidec_rpm/1
  slr_VHAL_RrEOPSpdSetNidec_rpm/1 -> RrEOPSpdSetNidec/1  "<VHAL_RrEOPSpdSetNidec_rpm>"
  True_VHAL_RrEOPSpdSetNidec_rpm/1 -> RrEOPSpdSetNidec/2
  [inp_CanValid_bus] -> slr1_2/1
  slr1_2/1 -> RrEOPSpdSetNidec/3  "<VINP_CANMsgValidMCUNR2_flg>"
  RrEOPSpdSetNidec/1 -> VINP_RrEOPSpdSetNidec_rpm/1  "VINP_RrEOPSpdSetNidec_rpm"
  RrEOPSpdSetNidec/2 -> Terminator_2/1
  [BHAL_outputs] -> slr_VHAL_RrFailcode1Nidec_enum/1
  slr_VHAL_RrFailcode1Nidec_enum/1 -> RrFailcode1Nidec/1  "<VHAL_RrFailcode1Nidec_enum>"
  True_VHAL_RrFailcode1Nidec_enum/1 -> RrFailcode1Nidec/2
  [inp_CanValid_bus] -> slr1_3/1
  slr1_3/1 -> RrFailcode1Nidec/3  "<VINP_CANMsgValidMCUNR2_flg>"
  RrFailcode1Nidec/1 -> VINP_RrFailcode1Nidec_enum/1  "VINP_RrFailcode1Nidec_enum"
  RrFailcode1Nidec/2 -> Terminator_3/1
  [BHAL_outputs] -> slr_VHAL_RrFailcode2Nidec_enum/1
  slr_VHAL_RrFailcode2Nidec_enum/1 -> RrFailcode2Nidec/1  "<VHAL_RrFailcode2Nidec_enum>"
  True_VHAL_RrFailcode2Nidec_enum/1 -> RrFailcode2Nidec/2
  [inp_CanValid_bus] -> slr1_4/1
  slr1_4/1 -> RrFailcode2Nidec/3  "<VINP_CANMsgValidMCUNR2_flg>"
  RrFailcode2Nidec/1 -> VINP_RrFailcode2Nidec_enum/1  "VINP_RrFailcode2Nidec_enum"
  RrFailcode2Nidec/2 -> Terminator_4/1
  [BHAL_outputs] -> slr_VHAL_RrFailcodehistory1Nidec_enum/1
  slr_VHAL_RrFailcodehistory1Nidec_enum/1 -> RrFailcodehistory1Nidec/1  "<VHAL_RrFailcodehistory1Nidec_enum>"
  True_VHAL_RrFailcodehistory1Nidec_enum/1 -> RrFailcodehistory1Nidec/2
  [inp_CanValid_bus] -> slr1_5/1
  slr1_5/1 -> RrFailcodehistory1Nidec/3  "<VINP_CANMsgValidMCUNR2_flg>"
  RrFailcodehistory1Nidec/1 -> VINP_RrFailcodehistory1Nidec_enum/1  "VINP_RrFailcodehistory1Nidec_enum"
  RrFailcodehistory1Nidec/2 -> Terminator_5/1
  [BHAL_outputs] -> slr_VHAL_RrFailcodehistory2Nidec_enum/1
  slr_VHAL_RrFailcodehistory2Nidec_enum/1 -> RrFailcodehistory2Nidec/1  "<VHAL_RrFailcodehistory2Nidec_enum>"
  True_VHAL_RrFailcodehistory2Nidec_enum/1 -> RrFailcodehistory2Nidec/2
  [inp_CanValid_bus] -> slr1_6/1
  slr1_6/1 -> RrFailcodehistory2Nidec/3  "<VINP_CANMsgValidMCUNR2_flg>"
  RrFailcodehistory2Nidec/1 -> VINP_RrFailcodehistory2Nidec_enum/1  "VINP_RrFailcodehistory2Nidec_enum"
  RrFailcodehistory2Nidec/2 -> Terminator_6/1
  [BHAL_outputs] -> slr_VHAL_RrLLCTempNidec_C/1
  slr_VHAL_RrLLCTempNidec_C/1 -> RrLLCTempNidec/1  "<VHAL_RrLLCTempNidec_C>"
  True_VHAL_RrLLCTempNidec_C/1 -> RrLLCTempNidec/2
  [inp_CanValid_bus] -> slr1_7/1
  slr1_7/1 -> RrLLCTempNidec/3  "<VINP_CANMsgValidMCUNR2_flg>"
  RrLLCTempNidec/1 -> VINP_RrLLCTempNidec_C/1  "VINP_RrLLCTempNidec_C"
  RrLLCTempNidec/2 -> Terminator_7/1
  [BHAL_outputs] -> slr_VHAL_RrLLCflowReqNidec_Lpmin/1
  slr_VHAL_RrLLCflowReqNidec_Lpmin/1 -> RrLLCflowReqNidec/1  "<VHAL_RrLLCflowReqNidec_Lpmin>"
  True_VHAL_RrLLCflowReqNidec_Lpmin/1 -> RrLLCflowReqNidec/2
  [inp_CanValid_bus] -> slr1_8/1
  slr1_8/1 -> RrLLCflowReqNidec/3  "<VINP_CANMsgValidMCUNR2_flg>"
  RrLLCflowReqNidec/1 -> VINP_RrLLCflowReqNidec_Lpmin/1  "VINP_RrLLCflowReqNidec_Lpmin"
  RrLLCflowReqNidec/2 -> Terminator_8/1
  [BHAL_outputs] -> slr_VHAL_RrMCUTempWarnNidec_enum/1
  slr_VHAL_RrMCUTempWarnNidec_enum/1 -> RrMCUTempWarnNidec/1  "<VHAL_RrMCUTempWarnNidec_enum>"
  True_VHAL_RrMCUTempWarnNidec_enum/1 -> RrMCUTempWarnNidec/2
  [inp_CanValid_bus] -> slr1_9/1
  slr1_9/1 -> RrMCUTempWarnNidec/3  "<VINP_CANMsgValidMCUNR2_flg>"
  RrMCUTempWarnNidec/1 -> VINP_RrMCUTempWarnNidec_enum/1  "VINP_RrMCUTempWarnNidec_enum"
  RrMCUTempWarnNidec/2 -> Terminator_9/1
  [BHAL_outputs] -> slr_VHAL_RrTMTempWarnNidec_enum/1
  slr_VHAL_RrTMTempWarnNidec_enum/1 -> RrTMTempWarnNidec/1  "<VHAL_RrTMTempWarnNidec_enum>"
  True_VHAL_RrTMTempWarnNidec_enum/1 -> RrTMTempWarnNidec/2
  [inp_CanValid_bus] -> slr1_10/1
  slr1_10/1 -> RrTMTempWarnNidec/3  "<VINP_CANMsgValidMCUNR2_flg>"
  RrTMTempWarnNidec/1 -> VINP_RrTMTempWarnNidec_enum/1  "VINP_RrTMTempWarnNidec_enum"
  RrTMTempWarnNidec/2 -> Terminator_10/1

== system inp/INP/CAN3/SignalCheck/MCU_N_R3 ==
  BHAL_outputs : Inport
  inp_CanValid_bus : Inport  Port=2
  RrMCU3HWVerNidec : FVT_lib/inp/can_signal_template  SystemSampleTime=-1  VariantActivationTime=update diagram  Latency=0  AutoFrameSizeCalculation=off
      link override defval: Value=KINP_RrMCU3HWVerNidec_enum_defval
      link override ovrdflg: Value=KINP_RrMCU3HWVerNidec_enum_ovrdflg
      link override ovrdval: Value=KINP_RrMCU3HWVerNidec_enum_ovrdval
  RrMCU3SWVerNidec : FVT_lib/inp/can_signal_template  SystemSampleTime=-1  VariantActivationTime=update diagram  Latency=0  AutoFrameSizeCalculation=off
      link override defval: Value=KINP_RrMCU3SWVerNidec_enum_defval
      link override ovrdflg: Value=KINP_RrMCU3SWVerNidec_enum_ovrdflg
      link override ovrdval: Value=KINP_RrMCU3SWVerNidec_enum_ovrdval
  Terminator_1 : Terminator
  Terminator_2 : Terminator
  True_VHAL_RrMCU3HWVerNidec_enum : Constant  Value=TRUE  OutDataTypeStr=boolean
  True_VHAL_RrMCU3SWVerNidec_enum : Constant  Value=TRUE  OutDataTypeStr=boolean
  slr1_1 : BusSelector  OutputSignals=VINP_CANMsgValidMCUNR3_flg
  slr1_2 : BusSelector  OutputSignals=VINP_CANMsgValidMCUNR3_flg
  slr_VHAL_RrMCU3HWVerNidec_enum : BusSelector  OutputSignals=VHAL_RrMCU3HWVerNidec_enum
  slr_VHAL_RrMCU3SWVerNidec_enum : BusSelector  OutputSignals=VHAL_RrMCU3SWVerNidec_enum
  VINP_RrMCU3HWVerNidec_enum : Outport
  VINP_RrMCU3SWVerNidec_enum : Outport  Port=2
  wires:
  BHAL_outputs/1 -> [BHAL_outputs]
  inp_CanValid_bus/1 -> [inp_CanValid_bus]
  [BHAL_outputs] -> slr_VHAL_RrMCU3HWVerNidec_enum/1
  slr_VHAL_RrMCU3HWVerNidec_enum/1 -> RrMCU3HWVerNidec/1  "<VHAL_RrMCU3HWVerNidec_enum>"
  True_VHAL_RrMCU3HWVerNidec_enum/1 -> RrMCU3HWVerNidec/2
  [inp_CanValid_bus] -> slr1_1/1
  slr1_1/1 -> RrMCU3HWVerNidec/3  "<VINP_CANMsgValidMCUNR3_flg>"
  RrMCU3HWVerNidec/1 -> VINP_RrMCU3HWVerNidec_enum/1  "VINP_RrMCU3HWVerNidec_enum"
  RrMCU3HWVerNidec/2 -> Terminator_1/1
  [BHAL_outputs] -> slr_VHAL_RrMCU3SWVerNidec_enum/1
  slr_VHAL_RrMCU3SWVerNidec_enum/1 -> RrMCU3SWVerNidec/1  "<VHAL_RrMCU3SWVerNidec_enum>"
  True_VHAL_RrMCU3SWVerNidec_enum/1 -> RrMCU3SWVerNidec/2
  [inp_CanValid_bus] -> slr1_2/1
  slr1_2/1 -> RrMCU3SWVerNidec/3  "<VINP_CANMsgValidMCUNR3_flg>"
  RrMCU3SWVerNidec/1 -> VINP_RrMCU3SWVerNidec_enum/1  "VINP_RrMCU3SWVerNidec_enum"
  RrMCU3SWVerNidec/2 -> Terminator_2/1

== system inp/INP/CAN3/SignalCheck/Shifter1 ==
  BHAL_outputs : Inport
  inp_CanValid_bus : Inport  Port=2
  Shifter1CSErr : FVT_lib/inp/can_signal_template  SystemSampleTime=-1  VariantActivationTime=update diagram  Latency=0  AutoFrameSizeCalculation=off
      link override defval: Value=KINP_Shifter1CSErr_flg_defval
      link override ovrdflg: Value=KINP_Shifter1CSErr_flg_ovrdflg
      link override ovrdval: Value=KINP_Shifter1CSErr_flg_ovrdval
  Shifter1RCErr : FVT_lib/inp/can_signal_template  SystemSampleTime=-1  VariantActivationTime=update diagram  Latency=0  AutoFrameSizeCalculation=off
      link override defval: Value=KINP_Shifter1RCErr_flg_defval
      link override ovrdflg: Value=KINP_Shifter1RCErr_flg_ovrdflg
      link override ovrdval: Value=KINP_Shifter1RCErr_flg_ovrdval
  ShifterCRC8 : FVT_lib/inp/can_signal_template  SystemSampleTime=-1  VariantActivationTime=update diagram  Latency=0  AutoFrameSizeCalculation=off
      link override defval: Value=KINP_ShifterCRC8_enum_defval
      link override ovrdflg: Value=KINP_ShifterCRC8_enum_ovrdflg
      link override ovrdval: Value=KINP_ShifterCRC8_enum_ovrdval
  ShifterFailsta : FVT_lib/inp/can_signal_template  SystemSampleTime=-1  VariantActivationTime=update diagram  Latency=0  AutoFrameSizeCalculation=off
      link override defval: Value=KINP_ShifterFailsta_enum_defval
      link override ovrdflg: Value=KINP_ShifterFailsta_enum_ovrdflg
      link override ovrdval: Value=KINP_ShifterFailsta_enum_ovrdval
  ShifterHandleCmd : FVT_lib/inp/can_signal_template  SystemSampleTime=-1  VariantActivationTime=update diagram  Latency=0  AutoFrameSizeCalculation=off
      link override defval: Value=KINP_ShifterHandleCmd_enum_defval
      link override ovrdflg: Value=KINP_ShifterHandleCmd_enum_ovrdflg
      link override ovrdval: Value=KINP_ShifterHandleCmd_enum_ovrdval
  ShifterRC : FVT_lib/inp/can_signal_template  SystemSampleTime=-1  VariantActivationTime=update diagram  Latency=0  AutoFrameSizeCalculation=off
      link override defval: Value=KINP_ShifterRC_enum_defval
      link override ovrdflg: Value=KINP_ShifterRC_enum_ovrdflg
      link override ovrdval: Value=KINP_ShifterRC_enum_ovrdval
  Terminator_{1..6} (6 alike) : Terminator
  True_VHAL_Shifter1CSErr_flg : Constant  Value=TRUE  OutDataTypeStr=boolean
  True_VHAL_Shifter1RCErr_flg : Constant  Value=TRUE  OutDataTypeStr=boolean
  True_VHAL_ShifterCRC8_enum : Constant  Value=TRUE  OutDataTypeStr=boolean
  True_VHAL_ShifterFailsta_enum : Constant  Value=TRUE  OutDataTypeStr=boolean
  True_VHAL_ShifterHandleCmd_enum : Constant  Value=TRUE  OutDataTypeStr=boolean
  True_VHAL_ShifterRC_enum : Constant  Value=TRUE  OutDataTypeStr=boolean
  slr1_{1..6} (6 alike) : BusSelector  OutputSignals=VINP_CANMsgValidShifter1_flg
  slr_VHAL_Shifter1CSErr_flg : BusSelector  OutputSignals=VHAL_Shifter1CSErr_flg
  slr_VHAL_Shifter1RCErr_flg : BusSelector  OutputSignals=VHAL_Shifter1RCErr_flg
  slr_VHAL_ShifterCRC8_enum : BusSelector  OutputSignals=VHAL_ShifterCRC8_enum
  slr_VHAL_ShifterFailsta_enum : BusSelector  OutputSignals=VHAL_ShifterFailsta_enum
  slr_VHAL_ShifterHandleCmd_enum : BusSelector  OutputSignals=VHAL_ShifterHandleCmd_enum
  slr_VHAL_ShifterRC_enum : BusSelector  OutputSignals=VHAL_ShifterRC_enum
  VINP_Shifter1CSErr_flg : Outport
  VINP_Shifter1RCErr_flg : Outport  Port=2
  VINP_ShifterCRC8_enum : Outport  Port=3
  VINP_ShifterFailsta_enum : Outport  Port=4
  VINP_ShifterHandleCmd_enum : Outport  Port=5
  VINP_ShifterRC_enum : Outport  Port=6
  wires:
  BHAL_outputs/1 -> [BHAL_outputs]
  inp_CanValid_bus/1 -> [inp_CanValid_bus]
  [BHAL_outputs] -> slr_VHAL_Shifter1CSErr_flg/1
  slr_VHAL_Shifter1CSErr_flg/1 -> Shifter1CSErr/1  "<VHAL_Shifter1CSErr_flg>"
  True_VHAL_Shifter1CSErr_flg/1 -> Shifter1CSErr/2
  [inp_CanValid_bus] -> slr1_1/1
  slr1_1/1 -> Shifter1CSErr/3  "<VINP_CANMsgValidShifter1_flg>"
  Shifter1CSErr/1 -> VINP_Shifter1CSErr_flg/1  "VINP_Shifter1CSErr_flg"
  Shifter1CSErr/2 -> Terminator_1/1
  [BHAL_outputs] -> slr_VHAL_Shifter1RCErr_flg/1
  slr_VHAL_Shifter1RCErr_flg/1 -> Shifter1RCErr/1  "<VHAL_Shifter1RCErr_flg>"
  True_VHAL_Shifter1RCErr_flg/1 -> Shifter1RCErr/2
  [inp_CanValid_bus] -> slr1_2/1
  slr1_2/1 -> Shifter1RCErr/3  "<VINP_CANMsgValidShifter1_flg>"
  Shifter1RCErr/1 -> VINP_Shifter1RCErr_flg/1  "VINP_Shifter1RCErr_flg"
  Shifter1RCErr/2 -> Terminator_2/1
  [BHAL_outputs] -> slr_VHAL_ShifterCRC8_enum/1
  slr_VHAL_ShifterCRC8_enum/1 -> ShifterCRC8/1  "<VHAL_ShifterCRC8_enum>"
  True_VHAL_ShifterCRC8_enum/1 -> ShifterCRC8/2
  [inp_CanValid_bus] -> slr1_3/1
  slr1_3/1 -> ShifterCRC8/3  "<VINP_CANMsgValidShifter1_flg>"
  ShifterCRC8/1 -> VINP_ShifterCRC8_enum/1  "VINP_ShifterCRC8_enum"
  ShifterCRC8/2 -> Terminator_3/1
  [BHAL_outputs] -> slr_VHAL_ShifterFailsta_enum/1
  slr_VHAL_ShifterFailsta_enum/1 -> ShifterFailsta/1  "<VHAL_ShifterFailsta_enum>"
  True_VHAL_ShifterFailsta_enum/1 -> ShifterFailsta/2
  [inp_CanValid_bus] -> slr1_4/1
  slr1_4/1 -> ShifterFailsta/3  "<VINP_CANMsgValidShifter1_flg>"
  ShifterFailsta/1 -> VINP_ShifterFailsta_enum/1  "VINP_ShifterFailsta_enum"
  ShifterFailsta/2 -> Terminator_4/1
  [BHAL_outputs] -> slr_VHAL_ShifterHandleCmd_enum/1
  slr_VHAL_ShifterHandleCmd_enum/1 -> ShifterHandleCmd/1  "<VHAL_ShifterHandleCmd_enum>"
  True_VHAL_ShifterHandleCmd_enum/1 -> ShifterHandleCmd/2
  [inp_CanValid_bus] -> slr1_5/1
  slr1_5/1 -> ShifterHandleCmd/3  "<VINP_CANMsgValidShifter1_flg>"
  ShifterHandleCmd/1 -> VINP_ShifterHandleCmd_enum/1  "VINP_ShifterHandleCmd_enum"
  ShifterHandleCmd/2 -> Terminator_5/1
  [BHAL_outputs] -> slr_VHAL_ShifterRC_enum/1
  slr_VHAL_ShifterRC_enum/1 -> ShifterRC/1  "<VHAL_ShifterRC_enum>"
  True_VHAL_ShifterRC_enum/1 -> ShifterRC/2
  [inp_CanValid_bus] -> slr1_6/1
  slr1_6/1 -> ShifterRC/3  "<VINP_CANMsgValidShifter1_flg>"
  ShifterRC/1 -> VINP_ShifterRC_enum/1  "VINP_ShifterRC_enum"
  ShifterRC/2 -> Terminator_6/1
